simulink subsystem "FTC"  (R2020b)
settings: Solver=VariableStepAuto  StartTime=0.0  StopTime=10.0  RelTol=1e-3
values from neighbouring files (symbols this model uses):
  g = (9.8)    (= 9.8)    [H250_LOEKnown_400HzParam.m]    (also in H250_LOEUnknown_400HzParam.m; H333_LOEKnown_400HzParam.m)
  J = (diag([0.0056 0.0056 0.0104]))    [H250_LOEKnown_400HzParam.m]    (also in H250_LOEUnknown_400HzParam.m; H333_LOEKnown_400HzParam.m = (diag([0.012 0.0120 0.02])))
  M = ([ 1          1          1         1 ... (first row only)    [H250_LOEKnown_400HzParam.m]    (also in H250_LOEUnknown_400HzParam.m; H333_LOEKnown_400HzParam.m)
  m = (0.700)    (= 0.7)    [H250_LOEKnown_400HzParam.m]    (also in H250_LOEUnknown_400HzParam.m = 0.752; H333_LOEKnown_400HzParam.m = 1.13)
  MY_ATT_P = Pixhawk_CSC.Parameter( {single(5), 'MY_ATT_P'}  )    [H250_LOEKnown_400HzParam.m]    (also in H250_LOEUnknown_400HzParam.m = Pixhawk_CSC.Parameter( {single(3), 'MY_ATT_P'}  ); H333_LOEKnown_400HzParam.m = Pixhawk_CSC.Parameter( {single(8), 'MY_ATT_P'}  ))
  MY_ATT_P_YAW = Pixhawk_CSC.Parameter( {single(0), 'MY_ATT_P_YAW'}  )    [H250_LOEKnown_400HzParam.m]    (also in H250_LOEUnknown_400HzParam.m = Pixhawk_CSC.Parameter( {single(0.0), 'MY_ATT_P_YAW'}  ); H333_LOEKnown_400HzParam.m)
  MY_K_CP = Pixhawk_CSC.Parameter({single(0.4), 'MY_K_CP'} )    [H250_LOEKnown_400HzParam.m]    (also in H250_LOEUnknown_400HzParam.m = Pixhawk_CSC.Parameter({single(0.7), 'MY_K_CP'} ))
  MY_POS_P = Pixhawk_CSC.Parameter( {single(0.8), 'MY_POS_P'}  )    [H250_LOEKnown_400HzParam.m]    (also in H250_LOEUnknown_400HzParam.m = Pixhawk_CSC.Parameter( {single(0.5), 'MY_POS_P'}  ); H333_LOEKnown_400HzParam.m = Pixhawk_CSC.Parameter( {single(0.5), 'MY_POS_P'}  ))
  MY_RATE_P = Pixhawk_CSC.Parameter( {single(14), 'MY_RATE_P'}  )    [H250_LOEKnown_400HzParam.m]    (also in H250_LOEUnknown_400HzParam.m; H333_LOEKnown_400HzParam.m = Pixhawk_CSC.Parameter( {single(12), 'MY_RATE_P'}  ))
  MY_RATE_P_YAW = Pixhawk_CSC.Parameter( {single(0.3), 'MY_RATE_P_YAW'}  )    [H250_LOEKnown_400HzParam.m]    (also in H250_LOEUnknown_400HzParam.m = Pixhawk_CSC.Parameter( {single(0.0), 'MY_RATE_P_YAW'}  ); H333_LOEKnown_400HzParam.m)
  MY_SAT_AD = Pixhawk_CSC.Parameter({single(0.15), 'MY_SAT_AD'} )    [H250_LOEKnown_400HzParam.m]    (also in H250_LOEUnknown_400HzParam.m = Pixhawk_CSC.Parameter({single(0.13), 'MY_SAT_AD'} ); H333_LOEKnown_400HzParam.m = Pixhawk_CSC.Parameter({single(0.13), 'MY_SAT_AD'} ))
  MY_TAU_P_A = Pixhawk_CSC.Parameter( {single(0), 'MY_TAU_P_A'}  )    [H250_LOEKnown_400HzParam.m]    (also in H250_LOEUnknown_400HzParam.m = Pixhawk_CSC.Parameter( {single(0.0), 'MY_TAU_P_A'}  ); H333_LOEKnown_400HzParam.m)
  MY_TAU_P_A_YAW = Pixhawk_CSC.Parameter( {single(0), 'MY_TAU_P_A_YAW'}  )    [H250_LOEKnown_400HzParam.m]    (also in H250_LOEUnknown_400HzParam.m; H333_LOEKnown_400HzParam.m)
  MY_TAU_P_P = Pixhawk_CSC.Parameter( {single(1.5), 'MY_TAU_P_P'}  )    [H250_LOEKnown_400HzParam.m]    (also in H250_LOEUnknown_400HzParam.m = Pixhawk_CSC.Parameter( {single(1.3), 'MY_TAU_P_P'}  ); H333_LOEKnown_400HzParam.m)
  MY_TAU_P_P_YAW = Pixhawk_CSC.Parameter( {single(0.1), 'MY_TAU_P_P_YAW'}  )    [H250_LOEKnown_400HzParam.m]    (also in H250_LOEUnknown_400HzParam.m; H333_LOEKnown_400HzParam.m)
  MY_VEL_P = Pixhawk_CSC.Parameter( {single(0.8), 'MY_VEL_P'}  )    [H250_LOEKnown_400HzParam.m]    (also in H250_LOEUnknown_400HzParam.m; H333_LOEKnown_400HzParam.m)
  MY_W_S = Pixhawk_CSC.Parameter({single(0), 'MY_W_S'} )    [H250_LOEKnown_400HzParam.m]
  MY_W_T = Pixhawk_CSC.Parameter({single(0), 'MY_W_T'} )    [H250_LOEKnown_400HzParam.m]
  T00 = single([m*g/4 m*g/4 m*g/4 m*g/4]')    [H250_LOEKnown_400HzParam.m]    (also in H250_LOEUnknown_400HzParam.m; H333_LOEKnown_400HzParam.m)
  Tf = 0.06    [H250_LOEKnown_400HzParam.m]    (also in H250_LOEUnknown_400HzParam.m; H333_LOEKnown_400HzParam.m)
  Tmotorbar = (0.035)    (= 0.035)    [H250_LOEKnown_400HzParam.m]    (also in H250_LOEUnknown_400HzParam.m = 0.032; H333_LOEKnown_400HzParam.m)
  Ts = 1/400    (= 0.0025)    [H250_LOEKnown_400HzParam.m]    (also in H250_LOEUnknown_400HzParam.m; H333_LOEKnown_400HzParam.m)
undefined symbols (not defined in the file or in its folder): MY_UL
libraries: discretizing x8, simulink x2, pixhawk_slib_uORB_RW x1
settings Model: Creator=kcx06  LastModifiedBy=kcx06

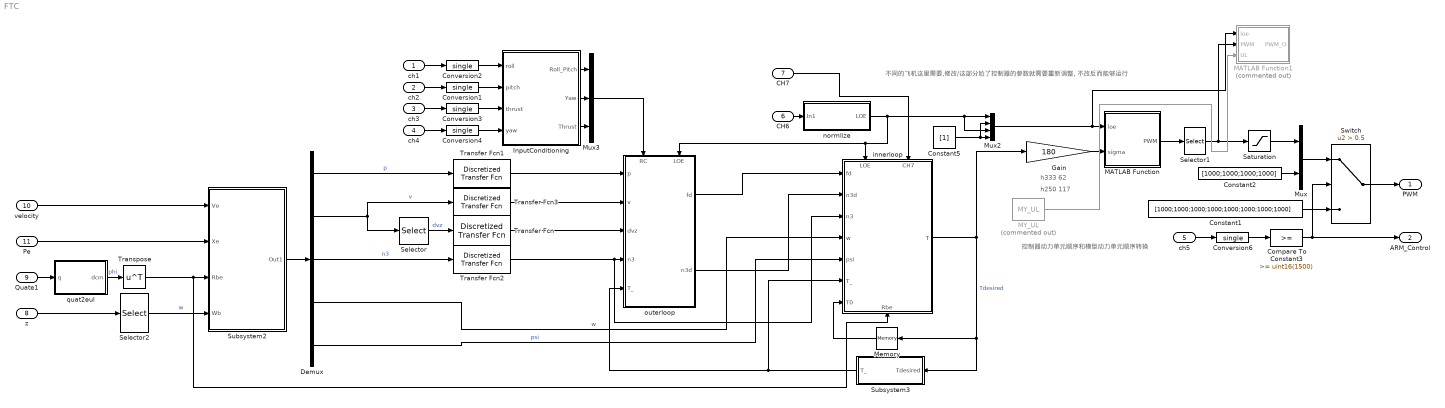
== system FTC ==
  note: h333 62
  note: h250 117
  note: 控制器动力单元顺序和模型动力单元顺序转换
  note: 不同的飞机这里需要,修改/这部分尬了控制器的参数就需要重新调整, 不改反而能够运行
  ch1 : Inport  OutDataTypeStr=uint16  PortDimensions=1
  ch2 : Inport  Port=2  OutDataTypeStr=uint16  PortDimensions=1
  ch3 : Inport  Port=3  OutDataTypeStr=uint16  PortDimensions=1
  ch4 : Inport  Port=4  OutDataTypeStr=uint16  PortDimensions=1
  ch5 : Inport  Port=5  OutDataTypeStr=uint16  PortDimensions=1  Interpolate=off
  CH6 : Inport  Port=6
  CH7 : Inport  Port=7
  z : Inport  Port=8
  Quate1 : Inport  Port=9
  velocity : Inport  Port=10
  Pe : Inport  Port=11
  Compare To Constant3 : simulink/Logic and Bit Operations/Compare To Constant  relop=>=  const=uint16(1500)  OutDataTypeStr=boolean
  Constant1 : Constant  Value=[1000;1000;1000;1000;1000;1000;1000;1000]  OutDataTypeStr=single
  Constant2 : Constant  Value=[1000;1000;1000;1000]  OutDataTypeStr=single
  Constant5 : Constant  Value=[1]  OutDataTypeStr=single
  Conversion{1..4,6} (5 alike) : DataTypeConversion  OutDataTypeStr=single
  Demux : Demux  Outputs=[3 3 3 3 1]
  Gain : Gain  Gain=180
  InputConditioning : Subsystem
  MATLAB Function : MATLAB Function  Description=1100-2000  TreatAsAtomicUnit=on
      settings: AttributesFormatString=1100-2000
  MATLAB Function1 : MATLAB Function  Commented=on  TreatAsAtomicUnit=on
  MY_UL : Constant  Commented=on  Value=MY_UL  OutDataTypeStr=single
  Memory : Memory  InitialCondition=T00
  Mux : Mux  Inputs=2
  Mux2 : Mux
  Mux3 : Mux  Inputs=3
  Saturation : Saturate  UpperLimit=1900  LowerLimit=900
  Selector : Selector  IndexMode=Zero-based  InputPortWidth=3  IndexOptions=Index vector (dialog)  Indices=[2]  OutputSizes=1
  Selector1 : Selector  IndexMode=Zero-based  InputPortWidth=4  IndexOptions=Index vector (dialog)  Indices=[0 2 3 1]  OutputSizes=1
  Selector2 : Selector  IndexMode=Zero-based  InputPortWidth=6  IndexOptions=Index vector (dialog)  Indices=[0 1 2]  OutputSizes=1
  Subsystem2 : Subsystem
  Subsystem3 : Subsystem
  Switch : Switch  Criteria=u2 > Threshold  Threshold=0.5
  Transfer Fcn : discretizing/Discretized Transfer Fcn  Numerator=[1 0]  Denominator=[Tf 1]  AbsTol=auto  SampleTime=Ts  method=zoh  Wc=1
      settings: SourceProductBaseCode=SL
  Transfer Fcn1 : discretizing/Discretized Transfer Fcn  Numerator=[1 ]  Denominator=[Tf 1]  AbsTol=auto  SampleTime=Ts  method=zoh  Wc=1
      link override Discrete Transfer Fcn: InitialStates=[0;0;0]
      settings: SourceProductBaseCode=SL
  Transfer Fcn2 : discretizing/Discretized Transfer Fcn  Numerator=[1 ]  Denominator=[Tf 1]  AbsTol=auto  SampleTime=Ts  method=zoh  Wc=1
      link override Discrete Transfer Fcn: InitialStates=[0;0;1]
      settings: SourceProductBaseCode=SL
  Transfer Fcn3 : discretizing/Discretized Transfer Fcn  Numerator=[1 ]  Denominator=[Tf 1]  AbsTol=auto  SampleTime=Ts  method=zoh  Wc=1
      link override Discrete Transfer Fcn: InitialStates=[0;0;0]
      settings: SourceProductBaseCode=SL
  Transpose : Math  Operator=transpose  SaturateOnIntegerOverflow=on
  innerloop : Subsystem
      settings: PortSchema="{\"entries\":[{\"content\":{\"sides\":[{\"content\":{\"connectorIds\":[\"In1\",\"In2\",\"In3\",\"In4\",\"In5\",\"In6\",\"In7\"]},\"type\":\"ConnectorPlacement.EquallySpacedRectSide\",\"uuid\":\"43c6e1bd-c98b-47b4-98da-f51fdffff433\"},{\"content\":{\"connectorIds\":[\"Out1\"],\"side\":\"RIGHT\"},\"type\":\"ConnectorPlacement.EquallySpacedRectSide\",\"uuid\":\"ac1c9532-9168-4bf4-8fed-08d3fdc16453\"},{\"content\":{\"connectorIds\":[\"In8\",\"In9\"],\"side\":\"TOP\"},\"type\":\"ConnectorPlacement.EquallySpacedRectSide\",\"uuid\":\"32774b13-030c-47c6-b846-fc6c0ce2dd6f\"},{\"content\":{\"connectorIds\":[\"In10\"],\"side\":\"BOTTOM\"},\"type\":\"ConnectorPlacement.EquallySpacedRectSide\",\"uuid\":\"153f8760-63e2-421b-ac58-9aae77834ac9\"}]},\"type\":\"ConnectorPlacement.EquallySpacedConnector\",\"uuid\":\"dd62421a-d766-429a-a161-5a0f77c5a7ba\"}],\"packageUris\":[\"http://schema.mathworks.com/mf0/Connector/R2020b\"],\"version\":\"1.0\"}"
  normlize : Subsystem
  outerloop : Subsystem
      settings: PortSchema="{\"entries\":[{\"content\":{\"sides\":[{\"content\":{\"connectorIds\":[\"In1\",\"In2\",\"In3\",\"In4\",\"In5\"]},\"type\":\"ConnectorPlacement.EquallySpacedRectSide\",\"uuid\":\"59983f3e-2daf-41bd-bc3f-074c85f4b2eb\"},{\"content\":{\"connectorIds\":[\"Out1\",\"Out2\"],\"side\":\"RIGHT\"},\"type\":\"ConnectorPlacement.EquallySpacedRectSide\",\"uuid\":\"6ee11e40-7870-4737-b9e6-fd7c25119100\"},{\"content\":{\"connectorIds\":[\"In6\",\"In7\"],\"side\":\"TOP\"},\"type\":\"ConnectorPlacement.EquallySpacedRectSide\",\"uuid\":\"847e9a02-4621-4cf8-a675-1479afa28be0\"}]},\"type\":\"ConnectorPlacement.EquallySpacedConnector\",\"uuid\":\"28981c41-e87e-4da3-ac2d-04a56d75ff2b\"}],\"packageUris\":[\"http://schema.mathworks.com/mf0/Connector/R2020b\"],\"version\":\"1.0\"}"
  quat2eul : MATLAB Function  TreatAsAtomicUnit=on
  PWM : Outport  PortDimensions=8  VectorParamsAs1DForOutWhenUnconnected=off
  ARM_Control : Outport  Port=2  PortDimensions=1  VectorParamsAs1DForOutWhenUnconnected=off
  wires:
  Compare To Constant3/1 -> ARM_Control/1, Switch/2
  Conversion4/1 -> InputConditioning/4(yaw)
  Saturation/1 -> Mux/1
  ch4/1 -> Conversion4/1
  ch2/1 -> Conversion1/1
  ch5/1 -> Conversion6/1
  Conversion1/1 -> InputConditioning/2(pitch)
  Conversion6/1 -> Compare To Constant3/1
  Conversion2/1 -> InputConditioning/1(roll)
  ch1/1 -> Conversion2/1
  ch3/1 -> Conversion3/1
  Constant2/1 -> Mux/2
  Mux/1 -> Switch/1
  Constant1/1 -> Switch/3
  innerloop/1(T) -> Gain/1, Memory/1, Subsystem3/1(Tdesired)  "Tdesired"
  Demux/5 -> innerloop/5(psi)  "psi"
  Memory/1 -> innerloop/7(T0)
  Selector/1 -> Transfer Fcn/1  "dvz"
  Demux/4 -> innerloop/4(w)  "w"
  Demux/2 -> Transfer Fcn3/1, Selector/1  "v"
  Selector1/1 -> MATLAB Function1/2(PWM), Saturation/1
  Gain/1 -> MATLAB Function/2(sigma)
  MATLAB Function/1(PWM) -> Selector1/1
  Subsystem2/1(Out1) -> Demux/1
  Selector2/1 -> Subsystem2/4(Wb)  "w"
  velocity/1 -> Subsystem2/1(Ve)
  Pe/1 -> Subsystem2/2(Xe)
  Quate1/1 -> quat2eul/1(q)
  Conversion3/1 -> InputConditioning/3(thrust)
  quat2eul/1(dcm) -> Transpose/1  "phi"
  outerloop/1(fd) -> innerloop/1(fd)
  Demux/1 -> Transfer Fcn1/1  "p"
  outerloop/2(n3d) -> innerloop/2(n3d)
  Subsystem3/1(T_) -> innerloop/6(T_), outerloop/5(T_)
  CH6/1 -> normlize/1(In1)
  normlize/1(LOE) -> Mux2/1, Mux2/3, innerloop/8(LOE), outerloop/7(LOE)
  Mux2/1 -> MATLAB Function/1(loe), MATLAB Function1/1(loe)
  Transfer Fcn/1 -> outerloop/3(dvz)
  Constant5/1 -> Mux2/4, Mux2/2
  Transpose/1 -> Subsystem2/3(Rbe), innerloop/10(Rbe)
  Demux/3 -> Transfer Fcn2/1  "n3"
  InputConditioning/1(Roll_Pitch) -> Mux3/1
  InputConditioning/2(Yaw) -> Mux3/2
  InputConditioning/3(Thrust) -> Mux3/3
  z/1 -> Selector2/1
  Mux3/1 -> outerloop/6(RC)
  Switch/1 -> PWM/1
  Transfer Fcn3/1 -> outerloop/2(v)
  Transfer Fcn1/1 -> outerloop/1(p)
  MY_UL/1 -> MATLAB Function1/3(UL)
  Transfer Fcn2/1 -> outerloop/4(n3), innerloop/3(n3)
  CH7/1 -> innerloop/9(CH7)

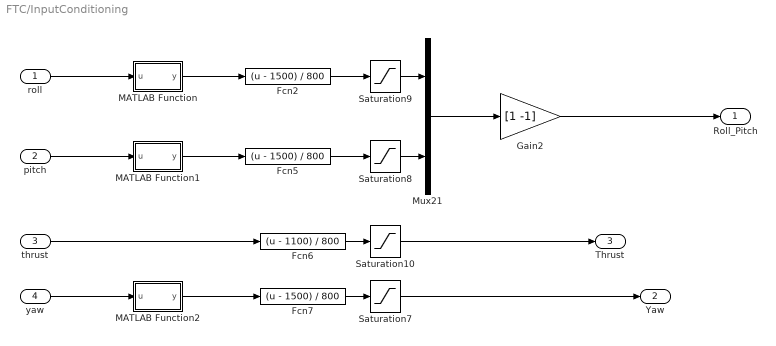
== system FTC/InputConditioning ==
  roll : Inport
  pitch : Inport  Port=2
  thrust : Inport  Port=3
  yaw : Inport  Port=4
  Fcn2 : Fcn  Expr=(u - 1500) / 800
  Fcn5 : Fcn  Expr=(u - 1500) / 800
  Fcn6 : Fcn  Expr=(u - 1100) / 800
  Fcn7 : Fcn  Expr=(u - 1500) / 800
  Gain2 : Gain  Gain=[1 -1]  OutDataTypeStr=Inherit: Inherit via back propagation
  MATLAB Function : MATLAB Function  TreatAsAtomicUnit=on
  MATLAB Function1 : MATLAB Function  TreatAsAtomicUnit=on
  MATLAB Function2 : MATLAB Function  TreatAsAtomicUnit=on
  Mux21 : Mux  Inputs=2
  Saturation10 : Saturate  UpperLimit=1  LowerLimit=0
  Saturation7 : Saturate  UpperLimit=1  LowerLimit=-1
  Saturation8 : Saturate  UpperLimit=1  LowerLimit=-1
  Saturation9 : Saturate  UpperLimit=1  LowerLimit=-1
  Roll_Pitch : Outport  VectorParamsAs1DForOutWhenUnconnected=off
  Yaw : Outport  Port=2  VectorParamsAs1DForOutWhenUnconnected=off
  Thrust : Outport  Port=3  VectorParamsAs1DForOutWhenUnconnected=off
  wires:
  yaw/1 -> MATLAB Function2/1(u)
  MATLAB Function/1(y) -> Fcn2/1
  MATLAB Function1/1(y) -> Fcn5/1
  roll/1 -> MATLAB Function/1(u)
  thrust/1 -> Fcn6/1
  MATLAB Function2/1(y) -> Fcn7/1
  pitch/1 -> MATLAB Function1/1(u)
  Fcn7/1 -> Saturation7/1
  Saturation9/1 -> Mux21/1
  Fcn5/1 -> Saturation8/1
  Fcn2/1 -> Saturation9/1
  Fcn6/1 -> Saturation10/1
  Saturation8/1 -> Mux21/2
  Mux21/1 -> Gain2/1
  Gain2/1 -> Roll_Pitch/1
  Saturation7/1 -> Yaw/1
  Saturation10/1 -> Thrust/1

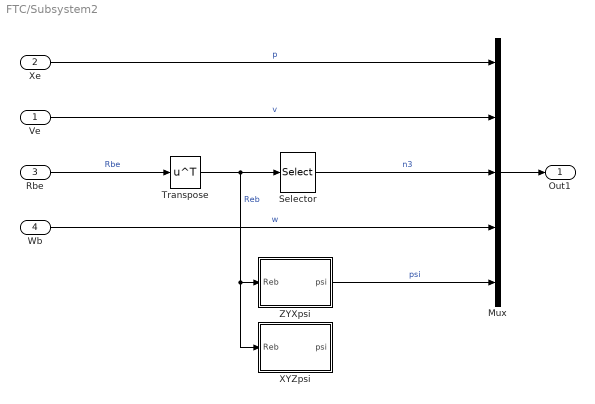
== system FTC/Subsystem2 ==
  Ve : Inport
  Xe : Inport  Port=2
  Rbe : Inport  Port=3
  Wb : Inport  Port=4
  Mux : Mux  Inputs=[3 3 3 3 1]
  Selector : Selector  NumberOfDimensions=2  IndexMode=Zero-based  InputPortWidth=3  IndexOptions=Select all,Index vector (dialog)  Indices=[1 3],2  OutputSizes=1,1
  Transpose : Math  Operator=transpose  SaturateOnIntegerOverflow=on
  XYZpsi : MATLAB Function  TreatAsAtomicUnit=on
  ZYXpsi : MATLAB Function  TreatAsAtomicUnit=on
  Out1 : Outport
  wires:
  ZYXpsi/1(psi) -> Mux/5  "psi"
  Wb/1 -> Mux/4  "w"
  Mux/1 -> Out1/1
  Selector/1 -> Mux/3  "n3"
  Transpose/1 -> Selector/1, ZYXpsi/1(Reb), XYZpsi/1(Reb)  "Reb"
  Rbe/1 -> Transpose/1  "Rbe"
  Ve/1 -> Mux/2  "v"
  Xe/1 -> Mux/1  "p"

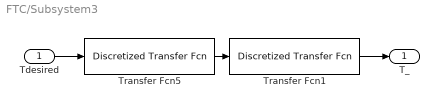
== system FTC/Subsystem3 ==
  Tdesired : Inport
  Transfer Fcn1 : discretizing/Discretized Transfer Fcn  Numerator=[1]  Denominator=[Tmotorbar 1]  AbsTol=auto  SampleTime=Ts  method=zoh  Wc=1
      settings: SourceProductBaseCode=SL
  Transfer Fcn5 : discretizing/Discretized Transfer Fcn  Numerator=[1]  Denominator=[Tf 1]  AbsTol=auto  SampleTime=Ts  method=zoh  Wc=1
      settings: SourceProductBaseCode=SL
  T_ : Outport
  wires:
  Tdesired/1 -> Transfer Fcn5/1
  Transfer Fcn1/1 -> T_/1
  Transfer Fcn5/1 -> Transfer Fcn1/1

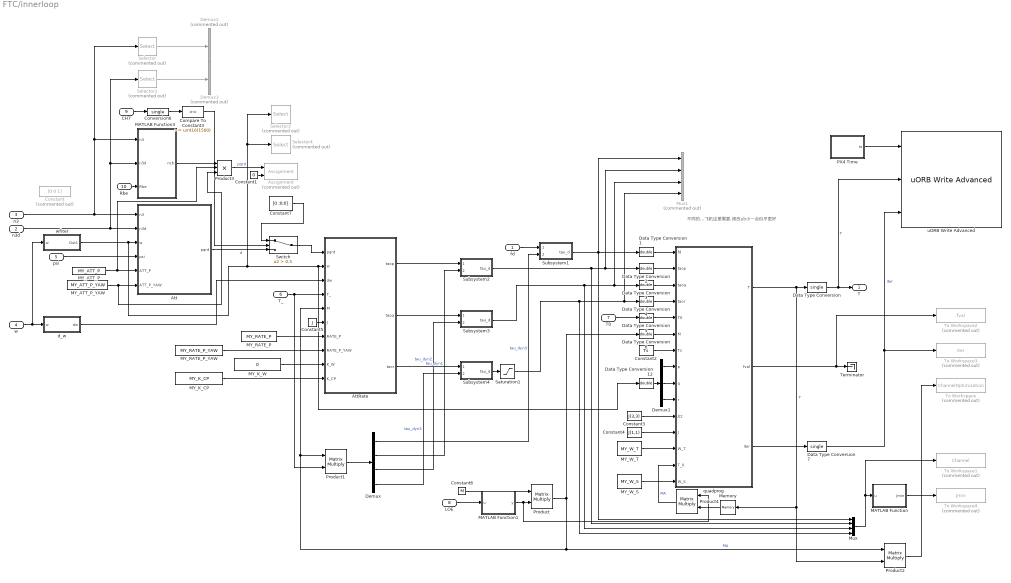
== system FTC/innerloop ==
  note: 不同的飞机这里需要,修改ub小一点似乎更好
  fd : Inport
  n3d : Inport  Port=2
  n3 : Inport  Port=3
  w : Inport  Port=4
  psi : Inport  Port=5
  T_ : Inport  Port=6
  T0 : Inport  Port=7
  LOE : Inport  Port=8
  CH7 : Inport  Port=9
  Rbe : Inport  Port=10
  Assignment : Assignment  Commented=on  DiagnosticForDimensions=Warning  IndexOptions=Index vector (dialog)  Indices=3  OutputSizes=1
  Att : MATLAB Function  TreatAsAtomicUnit=on
  AttRate : MATLAB Function  TreatAsAtomicUnit=on
  Compare To Constant3 : simulink/Logic and Bit Operations/Compare To Constant  relop=>=  const=uint16(1500)  OutDataTypeStr=boolean
  Constant : Constant  Commented=on  Value=[0 0 1]
  Constant1 : Constant  Value=0  OutDataTypeStr=single
  Constant2 : Constant  Value=Ts
  Constant3 : Constant  Value=J(3,3)
  Constant4 : Constant  Value=J(1,1)
  Constant5 : Constant  Value=J  OutDataTypeStr=single
  Constant6 : Constant  Value=M  OutDataTypeStr=single
  Constant7 : Constant  Value=[0 ;0;0]  OutDataTypeStr=single
  Conversion6 : DataTypeConversion  OutDataTypeStr=single
  Data Type Conversion : DataTypeConversion  OutDataTypeStr=single
  Data Type Conversion{1..6,12} (7 alike) : DataTypeConversion  OutDataTypeStr=double
  Data Type Conversion7 : DataTypeConversion  OutDataTypeStr=single
  Demux : Demux
  Demux1 : Demux  Outputs=3
  Demux2 : Demux  Commented=on  Outputs=2
  Demux3 : Demux  Commented=on  Outputs=2
  MATLAB Function : MATLAB Function  TreatAsAtomicUnit=on
  MATLAB Function1 : MATLAB Function  TreatAsAtomicUnit=on
  MATLAB Function3 : MATLAB Function  TreatAsAtomicUnit=on
  MY_ATT_P : Constant  Value=MY_ATT_P  SampleTime=-1
  MY_ATT_P_YAW : Constant  Value=MY_ATT_P_YAW  SampleTime=-1
  MY_K_CP : Constant  Value=MY_K_CP
  MY_K_W : Constant  Value=0
  MY_RATE_P : Constant  Value=MY_RATE_P
  MY_RATE_P_YAW : Constant  Value=MY_RATE_P_YAW
  MY_W_S : Constant  Value=MY_W_S  OutDataTypeStr=double
  MY_W_T : Constant  Value=MY_W_T  OutDataTypeStr=double
  Memory : Memory  InitialCondition=[0; 0; 0; 0]  InheritSampleTime=on
  Mux : Mux
  Mux1 : Mux  Commented=on
  PX4 Time : MATLAB Function  TreatAsAtomicUnit=on
  Product{,1..2,4} (4 alike) : Product  Multiplication=Matrix(*)
  Product3 : Product  Inputs=3
  Saturation1 : Saturate  UpperLimit=0.075  LowerLimit=-0.075
  Selector : Selector  Commented=on  InputPortWidth=3  IndexOptions=Index vector (dialog)  Indices=[1 2]  OutputSizes=1
  Selector1 : Selector  Commented=on  InputPortWidth=3  IndexOptions=Index vector (dialog)  Indices=[1 2]  OutputSizes=1
  Selector3 : Selector  Commented=on  InputPortWidth=3  IndexOptions=Index vector (dialog)  Indices=[1 2]  OutputSizes=1
  Selector4 : Selector  Commented=on  InputPortWidth=3  IndexOptions=Index vector (dialog)  Indices=[3]  OutputSizes=1
  Subsystem1 : Subsystem
  Subsystem2 : Subsystem
  Subsystem3 : Subsystem
  Subsystem4 : Subsystem
  Switch : Switch  Criteria=u2 > Threshold  Threshold=0.5
  Terminator : Terminator
  To Workspace : ToWorkspace  Commented=on  VariableName=ChannelOptimization  SaveFormat=Timeseries  SampleTime=-1
  To Workspace1 : ToWorkspace  Commented=on  VariableName=Channel  SaveFormat=Timeseries  SampleTime=-1
  To Workspace2 : ToWorkspace  Commented=on  VariableName=fval  SaveFormat=Timeseries  SampleTime=-1
  To Workspace3 : ToWorkspace  Commented=on  VariableName=iter  SaveFormat=Timeseries  SampleTime=-1
  To Workspace4 : ToWorkspace  Commented=on  VariableName=Jmin  SaveFormat=Timeseries  SampleTime=-1
  d_w : Subsystem
  quadprog : MATLAB Function  TreatAsAtomicUnit=on
  uORB Write Advanced : pixhawk_slib_uORB_RW/uORB Write Advanced  Ts=0  uORB_AdvtQueue=on  uORB_FieldEnabledArr="0  0  0  1  0  0  0  0  0  0  0"  uORB_Topic_str=0  uORB_Struct_DT="[1  1  1  1  1]"  BlockInputCount=5  uORB_StructParams="[\"voltage_v\",\"voltage_filtered_v\",\"current_a\",\"current_filtered_a\",\"remaining\"]"  uORB_PortSizes="[1  1  1  1]"  MsgSizeOf=0  MW_update=true
      settings: SourceProductName=Pixhawk Target Blocks
  wfiter : Subsystem
  T : Outport  PortDimensions=4
  wires:
  T0/1 -> Data Type Conversion5/1
  Product4/1 -> quadprog/14(T_0)  "MA"
  Constant7/1 -> Switch/1
  Switch/1 -> AttRate/1(pqrd)
  Compare To Constant3/1 -> Switch/2
  CH7/1 -> Conversion6/1
  Conversion6/1 -> Compare To Constant3/1
  MY_W_S/1 -> quadprog/15(W_S)
  Memory/1 -> Product4/2
  psi/1 -> Att/4(psi)
  MY_W_T/1 -> quadprog/13(W_T)
  Data Type Conversion12/1 -> Demux1/1
  Demux1/3 -> quadprog/10(r)
  Demux1/2 -> quadprog/9(q)
  Demux1/1 -> quadprog/8(p)
  Constant4/1 -> quadprog/12(J)
  Constant3/1 -> quadprog/11(Jzz)
  Constant2/1 -> quadprog/7(Ts)
  AttRate/3(taor) -> Subsystem4/1(tau_dynd)
  AttRate/2(taoq) -> Subsystem3/1(tau_dynd)
  AttRate/1(taop) -> Subsystem2/1(tau_dynd)
  MY_K_CP/1 -> AttRate/10(K_CP)
  MY_K_W/1 -> AttRate/9(K_W)
  Product1/1 -> Demux/1
  Constant1/1 -> Assignment/2
  Product3/1 -> Assignment/1  "pqrd"
  MATLAB Function3/1(ncb) -> Product3/1
  Rbe/1 -> MATLAB Function3/3(Rbe)
  n3d/1 -> Att/2(n3d), Selector1/1, MATLAB Function3/2(n3d)
  MATLAB Function/1(Jmin) -> To Workspace4/1
  Mux/1 -> MATLAB Function/1(u), To Workspace1/1
  Product2/1 -> To Workspace/1
  quadprog/3(iter) -> Data Type Conversion7/1
  Subsystem4/1(tau_d) -> Saturation1/1
  Subsystem3/1(tau_d) -> Mux/3, Data Type Conversion3/1, Mux1/3
  Subsystem2/1(tau_d) -> Mux/2, Data Type Conversion2/1, Mux1/2
  MY_ATT_P_YAW/1 -> Att/6(ATT_P_YAW), Product3/3
  MY_ATT_P/1 -> Att/5(ATT_P), Product3/2
  MY_RATE_P_YAW/1 -> AttRate/8(RATE_P_YAW)
  MY_RATE_P/1 -> AttRate/7(RATE_P)
  Data Type Conversion/1 -> T/1, uORB Write Advanced/2  "T"
  MATLAB Function1/1(y) -> Product/2, Product4/1
  Att/1(pqrd) -> Switch/3  "d"
  n3/1 -> MATLAB Function3/1(n3), Selector/1, Att/1(n3)
  Product/1 -> Data Type Conversion6/1, AttRate/5(M), Product1/1, Product2/1  "MA"
  LOE/1 -> MATLAB Function1/1(u)
  Saturation1/1 -> Mux/4, Data Type Conversion4/1, Mux1/4
  Demux/4 -> Subsystem4/2(tau_dyn)  "tau_dyn3"
  Demux/3 -> Subsystem3/2(tau_dyn)  "tau_dyn2"
  Demux/2 -> Subsystem2/2(tau_dyn)  "tau_dyn1"
  fd/1 -> Subsystem1/1(tau_dynd)
  Demux/1 -> Subsystem1/2(tau_dyn)  "tau_dyn3"
  Subsystem1/1(tau_d) -> Data Type Conversion1/1, Mux/1, Mux1/1
  Data Type Conversion6/1 -> quadprog/6(M)
  Data Type Conversion5/1 -> quadprog/5(T0)
  Data Type Conversion4/1 -> quadprog/4(taor)
  Data Type Conversion3/1 -> quadprog/3(taoq)
  Data Type Conversion2/1 -> quadprog/2(taop)
  Data Type Conversion1/1 -> quadprog/1(fd)
  quadprog/1(T) -> Data Type Conversion/1, Product2/2, Memory/1  "T"
  wfiter/1(Out1) -> Att/3(w), Selector3/1, Selector4/1, AttRate/2(w), Data Type Conversion12/1
  w/1 -> wfiter/1(w), d_w/1(w)
  quadprog/2(fval) -> Terminator/1, To Workspace2/1
  Constant6/1 -> Product/1
  Constant5/1 -> AttRate/6(J)
  T_/1 -> Product1/2, AttRate/4(T_)
  d_w/1(dw) -> AttRate/3(dw)
  PX4 Time/1(ts) -> uORB Write Advanced/1
  Selector/1 -> Demux2/1
  Selector1/1 -> Demux3/1
  Data Type Conversion7/1 -> uORB Write Advanced/3, To Workspace3/1  "iter"

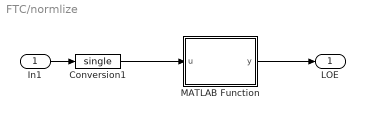
== system FTC/normlize ==
  In1 : Inport
  Conversion1 : DataTypeConversion  OutDataTypeStr=single
  MATLAB Function : MATLAB Function  TreatAsAtomicUnit=on
  LOE : Outport
  wires:
  MATLAB Function/1(y) -> LOE/1
  Conversion1/1 -> MATLAB Function/1(u)
  In1/1 -> Conversion1/1

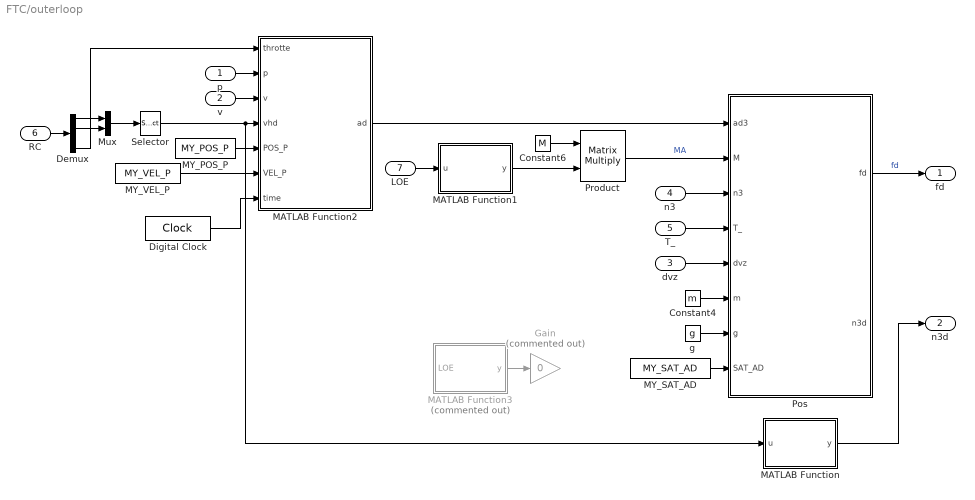
== system FTC/outerloop ==
  p : Inport
  v : Inport  Port=2
  dvz : Inport  Port=3
  n3 : Inport  Port=4
  T_ : Inport  Port=5
  RC : Inport  Port=6
  LOE : Inport  Port=7
  Constant4 : Constant  Value=m  OutDataTypeStr=single
  Constant6 : Constant  Value=M  OutDataTypeStr=single
  Demux : Demux
  Digital Clock : DigitalClock
  Gain : Gain  Commented=on  Gain=0
  MATLAB Function : MATLAB Function  TreatAsAtomicUnit=on
  MATLAB Function1 : MATLAB Function  TreatAsAtomicUnit=on
  MATLAB Function2 : MATLAB Function  TreatAsAtomicUnit=on
  MATLAB Function3 : MATLAB Function  Commented=on  TreatAsAtomicUnit=on
  MY_POS_P : Constant  Value=MY_POS_P
  MY_SAT_AD : Constant  Value=MY_SAT_AD
      settings: AttributesFormatString=|
      | 0.13
      | Default
  MY_VEL_P : Constant  Value=MY_VEL_P
  Mux : Mux  Inputs=2
  Pos : MATLAB Function  TreatAsAtomicUnit=on  SystemSampleTime=8*Ts
  Product : Product  Multiplication=Matrix(*)
  Selector : Selector  IndexMode=Zero-based  InputPortWidth=2  IndexOptions=Index vector (dialog)  Indices=[1 0]  OutputSizes=1
  g : Constant  Value=g  OutDataTypeStr=single
  fd : Outport
  n3d : Outport  Port=2
  wires:
  MATLAB Function3/1(y) -> Gain/1
  MATLAB Function2/1(ad) -> Pos/1(ad3)
  Digital Clock/1 -> MATLAB Function2/7(time)
  MY_SAT_AD/1 -> Pos/8(SAT_AD)
  MY_POS_P/1 -> MATLAB Function2/5(POS_P)
  MY_VEL_P/1 -> MATLAB Function2/6(VEL_P)
  Selector/1 -> MATLAB Function2/4(vhd), MATLAB Function/1(u)
  Mux/1 -> Selector/1
  Demux/2 -> Mux/2
  Demux/1 -> Mux/1
  v/1 -> MATLAB Function2/3(v)
  Demux/4 -> MATLAB Function2/1(throtte)
  RC/1 -> Demux/1
  Product/1 -> Pos/2(M)  "MA"
  Constant6/1 -> Product/1
  LOE/1 -> MATLAB Function1/1(u)
  MATLAB Function1/1(y) -> Product/2
  n3/1 -> Pos/3(n3)
  p/1 -> MATLAB Function2/2(p)
  g/1 -> Pos/7(g)
  Constant4/1 -> Pos/6(m)
  T_/1 -> Pos/4(T_)
  Pos/1(fd) -> fd/1  "fd"
  dvz/1 -> Pos/5(dvz)
  MATLAB Function/1(y) -> n3d/1

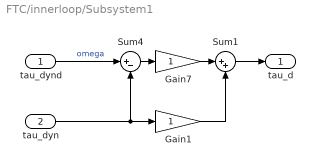
== system FTC/innerloop/Subsystem1 ==
  tau_dynd : Inport
  tau_dyn : Inport  Port=2
  Gain1 : Gain
  Gain7 : Gain
  Sum1 : Sum  Inputs=|++
  Sum4 : Sum  Inputs=|+-
  tau_d : Outport
  wires:
  Gain1/1 -> Sum1/2
  tau_dyn/1 -> Sum4/2, Gain1/1
  Sum1/1 -> tau_d/1
  Sum4/1 -> Gain7/1
  Gain7/1 -> Sum1/1
  tau_dynd/1 -> Sum4/1  "omega"

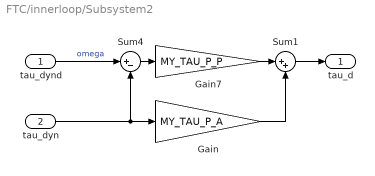
== system FTC/innerloop/Subsystem2 ==
  tau_dynd : Inport
  tau_dyn : Inport  Port=2
  Gain : Gain  Gain=MY_TAU_P_A
  Gain7 : Gain  Gain=MY_TAU_P_P
  Sum1 : Sum  Inputs=|++
  Sum4 : Sum  Inputs=|+-
  tau_d : Outport
  wires:
  Gain/1 -> Sum1/2
  tau_dynd/1 -> Sum4/1  "omega"
  Gain7/1 -> Sum1/1
  Sum4/1 -> Gain7/1
  Sum1/1 -> tau_d/1
  tau_dyn/1 -> Gain/1, Sum4/2

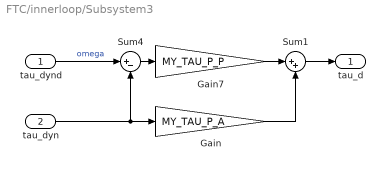
== system FTC/innerloop/Subsystem3 ==
  tau_dynd : Inport
  tau_dyn : Inport  Port=2
  Gain : Gain  Gain=MY_TAU_P_A
  Gain7 : Gain  Gain=MY_TAU_P_P
  Sum1 : Sum  Inputs=|++
  Sum4 : Sum  Inputs=|+-
  tau_d : Outport
  wires:
  tau_dyn/1 -> Sum4/2, Gain/1
  tau_dynd/1 -> Sum4/1  "omega"
  Gain/1 -> Sum1/2
  Sum1/1 -> tau_d/1
  Sum4/1 -> Gain7/1
  Gain7/1 -> Sum1/1

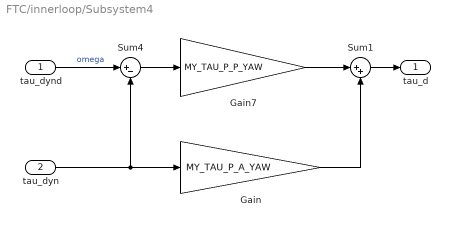
== system FTC/innerloop/Subsystem4 ==
  tau_dynd : Inport
  tau_dyn : Inport  Port=2
  Gain : Gain  Gain=MY_TAU_P_A_YAW
  Gain7 : Gain  Gain=MY_TAU_P_P_YAW
  Sum1 : Sum  Inputs=|++
  Sum4 : Sum  Inputs=|+-
  tau_d : Outport
  wires:
  Gain/1 -> Sum1/2
  tau_dynd/1 -> Sum4/1  "omega"
  Gain7/1 -> Sum1/1
  Sum4/1 -> Gain7/1
  Sum1/1 -> tau_d/1
  tau_dyn/1 -> Gain/1, Sum4/2

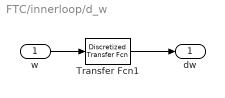
== system FTC/innerloop/d_w ==
  w : Inport
  Transfer Fcn1 : discretizing/Discretized Transfer Fcn  Numerator=[1 0]  Denominator=[Tf 1]  AbsTol=auto  SampleTime=Ts  method=zoh  Wc=1
      settings: SourceProductBaseCode=SL
  dw : Outport
  wires:
  Transfer Fcn1/1 -> dw/1
  w/1 -> Transfer Fcn1/1

== system FTC/innerloop/wfiter ==
  w : Inport
  Transfer Fcn1 : discretizing/Discretized Transfer Fcn  Numerator=[1]  Denominator=[Tf 1]  AbsTol=auto  SampleTime=Ts  method=zoh  Wc=1
      settings: SourceProductBaseCode=SL
  Out1 : Outport
  wires:
  Transfer Fcn1/1 -> Out1/1
  w/1 -> Transfer Fcn1/1

== matlab function FTC/InputConditioning/MATLAB Function1 ==
  data: u input; y output
function y = fcn(u)

 if(u>1550)
    y=u;
 else
     if(u<1450)
     y=u;
     else
         y=single(1500);
     end
 end

== matlab function FTC/InputConditioning/MATLAB Function2 ==
  data: u input; y output
function y = fcn(u)

 if(u>1550)
    y=u;
 else
     if(u<1450)
     y=u;
     else
         y=single(1500);
     end
 end

== matlab function FTC/MATLAB Function ==
  data: loe input; PWM output; sigma input
function PWM = fcn(loe, sigma)
y = loe.*sigma + 1100;
PWM = y;

== matlab function FTC/outerloop/MATLAB Function1 ==
  data: u input; y output
function y = fcn(u)
y=diag([u,1,u,1]);

== matlab function FTC/outerloop/MATLAB Function2 ==
  data: throtte input; ad output; p input; v input; vhd input; POS_P input; VEL_P input; time input
function ad = fcn(throtte, p, v, vhd, POS_P, VEL_P, time)
persistent pd
if isempty(pd)
    pd = single(p);
end
% 
% pd = single([0; 0; -5]);
% if time>=15
%     pd = single([80;0;-5]);
% end
% if time>=40
%     pd = single([80;50;-5]);
% end
% if time>=50
%     pd = single([0;50;-5]);
% end
% if time>=80
%     pd = single([0;40;-5]);
% end

%% 高度通道
if throtte>=0.4&& throtte <=0.6
        vd3 = mysatsingle(POS_P * (pd(3) - p(3)), 2);
        ad3 = VEL_P * (vd3 - v(3));
else
    if throtte>0.6
        vd3 = -1;
        ad3 = VEL_P * (vd3 - v(3));
        pd(3) = p(3);
    else
        vd3 = 1;
        ad3 = VEL_P * (vd3 - v(3));
        pd(3) = p(3);
    end
end
%% 水平通道
if norm(vhd) <= 0.05%0.05
        vd12 = mysatsingle(POS_P * (pd(1:2) - p(1:2)), 5);
        ad12 = VEL_P * (vd12 - v(1:2));
else
        vd12 = mysatsingle(5*vhd, 2);%0.7
        ad12 = VEL_P * (vd12 - v(1:2));
        pd(1:2) = p(1:2);
end
ad = [ad12;ad3];
% ad = [vhd;ad3];

== matlab function FTC/outerloop/Pos ==
  data: ad3 input single size=[3,1]; M input; n3 input; T_ input; dvz input; m input single size=1; fd output single size=1; g input single size=1; n3d output single size=3; SAT_AD input
function [fd, n3d]  = fcn(ad3, M, n3,  T_, dvz, m, g, SAT_AD)
ad = mysatsingle(ad3, single(SAT_AD)*g);
n3d = ([single(0); single(0); g]-ad)/norm([single(0); single(0); g]-ad);
if n3d(3)==single(0)
    fd = single(0);
else
    fd = (-ad(3) + dvz)*m/n3(3)+M(1,:)*T_;
end

== matlab function FTC/Subsystem2/ZYXpsi ==
  data: Reb input; psi output
function psi = fcn(Reb)
psi = atan2(Reb(2,1), Reb(1,1));

== matlab function FTC/innerloop/Att ==
  data: n3 input single; n3d input single; w input single; psi input single; pqrd output single; ATT_P input single; ATT_P_YAW input single
function pqrd  = fcn(n3, n3d, w, psi, ATT_P, ATT_P_YAW)
%% 角度控制1
% h1 = n3(1);
% h2 = n3(2);
% h3 = n3(3);
% h1d = n3d(1);
% h2d = n3d(2);
% h3d = n3d(3);
% we = Reb*w;
% k1 = single(5);
% epqd = [0 -1/h3; 1/h3 0]*[k1*(h1d-h1)+h2*we(3);k1*(h2d-h2)-h1*we(3)];
% 
% psid = single(0);
% rd = k1*0.3*(psid - psi);
% 
% Rbe = Reb';
% erd = (rd - Rbe(3,1)*epqd(1) - Rbe(3,2)*epqd(2))/Rbe(3,3);
% 
% pqd = Rbe((1:2),:)*[epqd; erd];%计算出机体系下的pqd
% pqd = mysat(pqd,2);
% pqrd = [pqd;rd];
%% 角度控制2
e1  = n3(1) - n3d(1);
e2  = n3(2) - n3d(2); 
beta = atan2(e2,e1);

k1 = ATT_P;
pqd = [ -k1*sqrt(e1^2+e2^2)*sin(psi-beta);
             -k1*sqrt(e1^2+e2^2)*cos(psi-beta);];
pqd = mysatsingle(pqd,2);
psid = 0;
   rd = -k1*ATT_P_YAW*(psi-psid);
% rd = 0;
pqrd = [pqd;rd];

== matlab function FTC/innerloop/AttRate ==
  data: pqrd input; w input; dw input; T_ input; M input; J input; taop output; taoq output; taor output; RATE_P input; RATE_P_YAW input; K_W input; K_CP input
function [taop, taoq, taor] = fcn(pqrd, w, dw, T_, M, J, RATE_P, RATE_P_YAW, K_W, K_CP)
pqd = pqrd(1:2);
rd    = pqrd(3);
%% 角速率控制器计算
k2 = RATE_P;
taop =           J(1,1)*(k2*(pqd(1)-w(1))) + M(2,:)*T_ -J(1,1)*dw(1) - K_W*w(1) + K_CP*(J(2,2)-J(3,3))*w(2)*w(3);
taoq =           J(2,2)*(k2*(pqd(2)-w(2))) + M(3,:)*T_ -J(2,2)*dw(2) - K_W*w(2) + K_CP*(J(3,3)-J(1,1))*w(1)*w(3);
taor  = mysatsingle(J(3,3)*k2*RATE_P_YAW*(rd-w(3)) + M(4,:)*T_ -J(3,3)*dw(3),20.0);

== matlab function FTC/innerloop/MATLAB Function1 ==
  data: u input; y output
function y = fcn(u)
y=diag([u,1,u,1]);

== matlab function FTC/innerloop/quadprog ==
  data: fd input double; taop input double; taoq input double; taor input double; T output double; T0 input double; M input double; fval output double; iter output; Ts input; p input; q input; r input; Jzz input; J input; W_T input; T_0 input; W_S input
function [T,fval, iter] = fcn(fd, taop, taoq, taor, T0, M, Ts, p, q, r, Jzz, J, W_T, T_0, W_S)
%% 求解
% T_0表示上一时刻控制分配
% T0表示上一时刻估计的电机输出
vd = [fd; taop; taoq; taor];
W=diag([1 100 100 0.01]);% W=diag([1 20 20 0.9]);
w_T = W_T;% 最小化输出权重
w_S = W_S;% 平滑因子权重
H = M'*W*M + diag([w_T w_T w_T w_T]) + diag([w_S w_S w_S w_S]);
f = -(vd'*W*M + w_T*[0,0,0,0] + w_S*T_0')';
% Td = B*vd;
lb  = [0 0 0 0]';
% ub  = [8.5 8.5 8.5 8.5]';%h250 8.5 8.5 8.5 8.5 %h333 16
ub  = [5 5 5 5]';

% if (max(B*vd)>3)||(min(B*vd)<0)
    options = optimoptions(@quadprog,'Algorithm','active-set','MaxIterations',10);

    [T,fval,~,output] = quadprog(H, f, [], [], [], [], lb, ub, T0, options);
     iter = output.iterations;
% else
%     T = B*vd;
%     fval = 0;
% end

== matlab function FTC/quat2eul ==
  data: q input single; dcm output single
function dcm  = quat2eul(q)
% Conversion from Quaternion to Euler angles based on the PX4 Firmware
% v1.6.5 release.
% 
% Quaternion -> DCM -> Euler Angles
% INPUT:
%   q: Quaternion vector of the format: (a + bi + cj + dk)
% OUTPUT:
%   [phi,theta,psi]: Euler angles in radians.
% 
 if norm(q)~=0
    a = q(1);
    b = q(2);
    c = q(3);
    d = q(4);

    aSq = a*a;
    bSq = b*b;
    cSq = c*c;
    dSq = d*d;

    d_pi2 = pi/2;

    % quaternion_to_dcm
    dcm00 = aSq + bSq - cSq - dSq;
    dcm01 = 2*(b*c - a*d);
    dcm02 = 2*(a*c + b*d);
    dcm10 = 2*(b*c + a*d);
    dcm11 = aSq - bSq + cSq - dSq;
    dcm12 = 2*(c*d - a*b);
    dcm20 = 2*(b*d - a*c);
    dcm21 = 2*(a*b + c*d);
    dcm22 = aSq - bSq - cSq + dSq;
    dcm=[dcm00 dcm01 dcm02;
              dcm10 dcm11 dcm12;
              dcm20 dcm21  dcm22];
 else
     dcm = single(eye(3,3));
 end
    % dcm_to_euler

== matlab function FTC/innerloop/PX4 Time ==
  data: ts output
function ts  = fcn
% coder.cinclude('drivers/drv_hrt.h');
persistent count
if isempty(count)
    count = 0;
end

hrt = 0;
if coder.target('Rtw')
    hrt = coder.ceval('hrt_absolute_time');
else
    hrt = count;
end
ts = hrt;% us

count = count + 1;

== matlab function FTC/innerloop/MATLAB Function ==
  data: u input; Jmin output
function Jmin = fcn(u)
W=diag([1 20 20 0.9]);
Jmin = -0.5*u'*W*u;

== matlab function FTC/Subsystem2/XYZpsi ==
  data: Reb input; psi output
function psi = fcn(Reb)
psi = atan2(-Reb(1,2), Reb(1,1));

== matlab function FTC/outerloop/MATLAB Function ==
  data: u input single; y output single
function y = fcn(u)
y = [-u/6; 1]/norm([-u/6; 1]);

== matlab function FTC/normlize/MATLAB Function ==
  data: u input; y output
function y = fcn(u)
if u<1400
    y = single(1);
else
    if u>1800
        y = single(0);
    else
        y = single(0.25);
    end
end

== matlab function FTC/MATLAB Function1 ==
  data: loe input; PWM_O output single; PWM input single; UL input single
function PWM_O = fcn(loe,PWM,UL)

PWM_OUT = single([0 0 0 0]);

if loe(1)<0.2
    PWM_ul = UL;%1145
else
    PWM_ul = single(900);
end

if PWM(1)>1900
    PWM_OUT(1) = single(1900);
else
    if PWM(1)<PWM_ul
        PWM_OUT(1) = PWM_ul;
    else
        PWM_OUT(1) = PWM(1);
    end
end

if PWM(2)>1900
    PWM_OUT(2) = single(1900);
else
    if PWM(2)<PWM_ul
        PWM_OUT(2) = PWM_ul;
    else
        PWM_OUT(2) = PWM(2);
    end
end

if PWM(3)>1900
    PWM_OUT(3) = single(1900);
else
    if PWM(3)<PWM_ul
        PWM_OUT(3) = PWM_ul;
    else
        PWM_OUT(3) = PWM(3);
    end
end

if PWM(4)>1900
    PWM_OUT(4) = single(1900);
else
    if PWM(4)<PWM_ul
        PWM_OUT(4) = PWM_ul;
    else
        PWM_OUT(4) = PWM(4);
    end
end

PWM_O = PWM_OUT;

== matlab function FTC/outerloop/MATLAB Function3 ==
  data: LOE input; y output
function y = fcn(LOE)
persistent n
if isempty(n)
    n = 0;
end

% if LOE<0.5
    n = n+1;
% end

if n==500
    n=0;
end

if n >= 450
    y = [1 0];
else
   y = [0 0];
end

== matlab function FTC/InputConditioning/MATLAB Function ==
  data: u input; y output
function y = fcn(u)

 if(u>1550)
    y=u;
 else
     if(u<1450)
     y=u;
     else
         y=single(1500);
     end
 end

== matlab function FTC/innerloop/MATLAB Function3 ==
  data: n3 input; ncb output; n3d input; Rbe input
function ncb = fcn(n3, n3d, Rbe)
nc = cross(n3, n3d);
ncb  = Rbe*nc;
